simulink model "experiment_toplevel_with_tail"  (R2016a)
settings: Solver=ode15s  StartTime=0.0  StopTime=8  MaxStep=1e-2  RelTol=1e-4
PreLoadFcn:
  | minitaurParameters
values from neighbouring files (symbols this model uses):
  angular_ctrl_d = 1    [minitaurParameters.m]
  angular_ctrl_i = 1    [minitaurParameters.m]
  angular_ctrl_p = 100    [minitaurParameters.m]
  enc_zero_IA = -1.25*pi    (= -3.92699081699)    [minitaurParameters.m]
  enc_zero_IB = -0.25*pi    (= -0.785398163397)    [minitaurParameters.m]
  enc_zero_IIA = 1.25*pi    (= 3.92699081699)    [minitaurParameters.m]
  enc_zero_IIB = 1.25*pi    (= 3.92699081699)    [minitaurParameters.m]
  enc_zero_IIIA = 0.5*pi    (= 1.57079632679)    [minitaurParameters.m]
  enc_zero_IIIB = 1.5*pi    (= 4.71238898038)    [minitaurParameters.m]
  enc_zero_IVA = -0.25*pi    (= -0.785398163397)    [minitaurParameters.m]
  enc_zero_IVB = 0.5*pi    (= 1.57079632679)    [minitaurParameters.m]
  enc_zero_tail = 0    [minitaurParameters.m]
  fore_lag = fore_lag_vals(j)    [experiment1.m]    (also in experiment1_parfor_accelerator.m = 0; minitaurParameters.m = 0.45)
  ground_frame_depth = 0.5    [minitaurParameters.m]
  ground_length = 100    [minitaurParameters.m]
  ground_width = 10    [minitaurParameters.m]
  init_theta_IA = -pi/4    (= -0.785398163397)    [minitaurParameters.m]
  init_theta_IB = pi/4    (= 0.785398163397)    [minitaurParameters.m]
  init_theta_IIA = -pi/4    (= -0.785398163397)    [minitaurParameters.m]
  init_theta_IIB = pi/4    (= 0.785398163397)    [minitaurParameters.m]
  init_theta_IIIA = -pi/4    (= -0.785398163397)    [minitaurParameters.m]
  init_theta_IIIB = pi/4    (= 0.785398163397)    [minitaurParameters.m]
  init_theta_IVA = -pi/4    (= -0.785398163397)    [minitaurParameters.m]
  init_theta_IVB = pi/4    (= 0.785398163397)    [minitaurParameters.m]
  init_theta_tail = 0    [minitaurParameters.m]
  l1 = 100e-3    (= 0.1)    [minitaurParameters.m]
  l2 = 200e-3    (= 0.2)    [minitaurParameters.m]
  leg_joint_radius = 3e-3    (= 0.003)    [minitaurParameters.m]
  lr_sync = 1    [experiment1.m]    (also in experiment1_parfor_accelerator.m; minitaurParameters.m = 0)
  model = 'experiment_toplevel'    [experiment1_parfor_accelerator.m]
  period = period_vals(i)    [experiment1.m]    (also in experiment1_parfor_accelerator.m = 1.5; minitaurParameters.m = 0.33)
  phi_0 = 0.5*asin(l1/l2)    [experiment1.m]    (also in experiment1_parfor_accelerator.m; minitaurParameters.m)
  r_0 = l2    [experiment1.m]    (also in experiment1_parfor_accelerator.m; minitaurParameters.m = 0.2)
  r_x = 0.3*l1    [experiment1.m]    (also in experiment1_parfor_accelerator.m = 0.5*l1; minitaurParameters.m = 0.05)
  r_y = 0.2*l1    [experiment1.m]    (also in experiment1_parfor_accelerator.m = 0.3*l1; minitaurParameters.m = 0.03)
  radial_ctrl_d = 1    [minitaurParameters.m]
  radial_ctrl_i = 1    [minitaurParameters.m]
  radial_ctrl_p = 80    [minitaurParameters.m]
  safety_limit = 10e-3    (= 0.01)    [minitaurParameters.m]
undefined symbols (not defined in the file or in its folder): Axis, Fn, minitaurParams, r_stance, r_swing, stance_frac, X, Y, Z
undefined symbols (not defined in the file): leg_joint_fric_bw, leg_joint_mu_k, leg_joint_mu_s, leg_joint_vel_thresh, motor_kt, motor_kv, motor_r, motor_torque_sat
libraries: sm_lib x488, fl_lib x132, nesl_utility x34, Contact_Forces_Lib x28, simulink x20
(part 14 of 14)

== system experiment_toplevel_with_tail/GR Minitaur/minitaur_motor_module_IVB/DYS_BLDC_86x10_BE8108_12/DYS_BLDC_86x10_BE8108_12_stator_1_RIGID ==
  ReferenceFrame : sm_lib/Frames and Transforms/Reference Frame
  Solid : sm_lib/Body Elements/Solid  InertiaType=Custom  Mass=minitaurParams.Solid(6).mass  MassUnits=kg  CenterOfMass=minitaurParams.Solid(6).CoM  CenterOfMassUnits=mm  MomentsOfInertia=minitaurParams.Solid(6).MoI  MomentsOfInertiaUnits=kg*mm^2  ProductsOfInertia=minitaurParams.Solid(6).PoI  ProductsOfInertiaUnits=kg*mm^2  DensityBased=on  Density=1000  DensityUnits=kg/(m^3)  DoExposeReferenceFrame=on  SerializedFrames=<Frames/>  GraphicType=FromGeometry  MarkerShape=Sphere  MarkerSize=10  GraphicVisPropType=SimpleVisualProperties  GraphicDiffuseColor=minitaurParams.Solid(6).color  GraphicSpecularColor=[0.5 0.5 0.5 1.0]  GraphicAmbientColor=[0.15 0.15 0.15 1.0]  GraphicEmissiveColor=[0.0 0.0 0.0 1.0]  GraphicShininess=75  GraphicOpacity=minitaurParams.Solid(6).opacity  GeometryShape=FromFile  RectangleSize=[1 1]  RectangleSizeUnits=m  BrickDimensions=[1 1 1]  BrickDimensionUnits=m  CylinderRadius=1  CylinderRadiusUnits=m  CylinderLength=1  CylinderLengthUnits=m  SphereRadius=1  SphereRadiusUnits=m  EllipsoidRadii=[1 1 1]  EllipsoidRadiiUnits=m  ExtrusionCrossSection=[1 1; -1 1; -1 -1; 1 -1]  ExtrusionCrossSectionUnits=m  ExtrusionLength=1  ExtrusionLengthUnits=m  PolygonNumSides=3  PolygonOuterRadius=1  PolygonOuterRadiusUnits=m  ExtGeomFileType=STEP  ExtGeomFileName=model/DYS-BLDC-86x10-BE8108-12-stator_Default_sldprt.STEP  ExtGeomFileUnits=m  RevolutionCrossSection=[1 1; 1 -1; 2 -1; 2 1]  RevolutionCrossSectionUnits=m  RevolutionExtent=Full  RevolutionAngle=180  RevolutionAngleUnits=deg
  Transform : sm_lib/Frames and Transforms/Rigid Transform  TranslationMethod=Cartesian  TranslationLengthUnit=mm  TranslationStandardAxis=+Z  TranslationStandardOffset=0  TranslationCartesianOffset=minitaurParams.RigidTransform(17).translation  TranslationROffset=0  TranslationROffsetUnits=m  TranslationZOffset=0  TranslationZOffsetUnits=m  TranslationThetaOffset=0  TranslationThetaOffsetUnits=deg  RotationMethod=ArbitraryAxis  RotationAngleUnits=rad  RotationStandardAxis=+Z  RotationAngle=minitaurParams.RigidTransform(17).angle  RotationArbitraryAxis=minitaurParams.RigidTransform(17).axis  FollAlignAxisA=+X  BaseAlignAxisA=+Y  FollAlignAxisB=+Y  BaseAlignAxisB=+Z  RotationSequenceAxes=FollowerAxes  RotationSequence=XYX  RotationSequenceAngles=[0 0 0]  RotationSequenceAnglesUnits=deg  RotationMatrix=[1 0 0; 0 1 0; 0 0 1]
  Transform1 : sm_lib/Frames and Transforms/Rigid Transform  TranslationMethod=Cartesian  TranslationLengthUnit=mm  TranslationStandardAxis=+Z  TranslationStandardOffset=0  TranslationCartesianOffset=minitaurParams.RigidTransform(19).translation  TranslationROffset=0  TranslationROffsetUnits=m  TranslationZOffset=0  TranslationZOffsetUnits=m  TranslationThetaOffset=0  TranslationThetaOffsetUnits=deg  RotationMethod=ArbitraryAxis  RotationAngleUnits=rad  RotationStandardAxis=+Z  RotationAngle=minitaurParams.RigidTransform(19).angle  RotationArbitraryAxis=minitaurParams.RigidTransform(19).axis  FollAlignAxisA=+X  BaseAlignAxisA=+Y  FollAlignAxisB=+Y  BaseAlignAxisB=+Z  RotationSequenceAxes=FollowerAxes  RotationSequence=XYX  RotationSequenceAngles=[0 0 0]  RotationSequenceAnglesUnits=deg  RotationMatrix=[1 0 0; 0 1 0; 0 0 1]
  Transform2 : sm_lib/Frames and Transforms/Rigid Transform  TranslationMethod=Cartesian  TranslationLengthUnit=mm  TranslationStandardAxis=+Z  TranslationStandardOffset=0  TranslationCartesianOffset=minitaurParams.RigidTransform(26).translation  TranslationROffset=0  TranslationROffsetUnits=m  TranslationZOffset=0  TranslationZOffsetUnits=m  TranslationThetaOffset=0  TranslationThetaOffsetUnits=deg  RotationMethod=ArbitraryAxis  RotationAngleUnits=rad  RotationStandardAxis=+Z  RotationAngle=minitaurParams.RigidTransform(26).angle  RotationArbitraryAxis=minitaurParams.RigidTransform(26).axis  FollAlignAxisA=+X  BaseAlignAxisA=+Y  FollAlignAxisB=+Y  BaseAlignAxisB=+Z  RotationSequenceAxes=FollowerAxes  RotationSequence=XYX  RotationSequenceAngles=[0 0 0]  RotationSequenceAnglesUnits=deg  RotationMatrix=[1 0 0; 0 1 0; 0 0 1]
  Transform3 : sm_lib/Frames and Transforms/Rigid Transform  TranslationMethod=Cartesian  TranslationLengthUnit=mm  TranslationStandardAxis=+Z  TranslationStandardOffset=0  TranslationCartesianOffset=minitaurParams.RigidTransform(62).translation  TranslationROffset=0  TranslationROffsetUnits=m  TranslationZOffset=0  TranslationZOffsetUnits=m  TranslationThetaOffset=0  TranslationThetaOffsetUnits=deg  RotationMethod=ArbitraryAxis  RotationAngleUnits=rad  RotationStandardAxis=+Z  RotationAngle=minitaurParams.RigidTransform(62).angle  RotationArbitraryAxis=minitaurParams.RigidTransform(62).axis  FollAlignAxisA=+X  BaseAlignAxisA=+Y  FollAlignAxisB=+Y  BaseAlignAxisB=+Z  RotationSequenceAxes=FollowerAxes  RotationSequence=XYX  RotationSequenceAngles=[0 0 0]  RotationSequenceAnglesUnits=deg  RotationMatrix=[1 0 0; 0 1 0; 0 0 1]
  F2 : PMIOPort  Port=1  Side=Left
  F3 : PMIOPort  Port=2  Side=Left
  F : PMIOPort  Port=3  Side=Left
  F1 : PMIOPort  Port=4  Side=Right
  connections:
  ReferenceFrame/RConn1 -- Solid/RConn1 -- Transform/LConn1 -- Transform1/LConn1 -- Transform2/LConn1 -- Transform3/LConn1
  Transform/RConn1 -- F/RConn1
  Transform1/RConn1 -- F1/RConn1
  Transform2/RConn1 -- F2/RConn1
  Transform3/RConn1 -- F3/RConn1

== system experiment_toplevel_with_tail/GR Minitaur/minitaur_motor_module_Tail/DYS_BLDC_86x10_BE8108_12/BLDC Model ==
  Desired Torque  [Nm] : Inport
  Velocity [rad/s] : Inport  Port=2
  Constant : Constant  Value=torque_sat
  Constant1 : Constant  Value=-torque_sat
  Gain : Gain  Gain=1/kt
  Gain1 : Gain  Gain=r
  Math Function : Math  Operator=square  SaturateOnIntegerOverflow=on
  Saturation Dynamic : simulink/Discontinuities/Saturation Dynamic  OutMin=[]  OutMax=[]  OutDataTypeStr=Inherit: Same as second input  OutDataType=fixdt(1, 16)  OutScaling=2^-10  DoSatur=off
  Terminator : Terminator
  Transfer Fcn : TransferFcn  Denominator=[timeconst 1]
  Torque [N*m] : Outport
  Ploss [W] : Outport  Port=2
  wires:
  Desired Torque  [Nm]/1 -> Transfer Fcn/1
  Math Function/1 -> Gain1/1
  Gain/1 -> Math Function/1
  Gain1/1 -> Ploss [W]/1
  Velocity [rad/s]/1 -> Terminator/1
  Transfer Fcn/1 -> Saturation Dynamic/2
  Saturation Dynamic/1 -> Gain/1, Torque [N*m]/1
  Constant/1 -> Saturation Dynamic/1
  Constant1/1 -> Saturation Dynamic/3

== system experiment_toplevel_with_tail/GR Minitaur/minitaur_motor_module_Tail/DYS_BLDC_86x10_BE8108_12/DYS_BLDC_86x10_BE8108_12_rotor_1_RIGID ==
  ReferenceFrame : sm_lib/Frames and Transforms/Reference Frame
  Solid : sm_lib/Body Elements/Solid  InertiaType=Custom  Mass=minitaurParams.Solid(7).mass  MassUnits=kg  CenterOfMass=minitaurParams.Solid(7).CoM  CenterOfMassUnits=mm  MomentsOfInertia=minitaurParams.Solid(7).MoI  MomentsOfInertiaUnits=kg*mm^2  ProductsOfInertia=minitaurParams.Solid(7).PoI  ProductsOfInertiaUnits=kg*mm^2  DensityBased=on  Density=1000  DensityUnits=kg/(m^3)  DoExposeReferenceFrame=on  SerializedFrames=<Frames/>  GraphicType=FromGeometry  MarkerShape=Sphere  MarkerSize=10  GraphicVisPropType=SimpleVisualProperties  GraphicDiffuseColor=minitaurParams.Solid(7).color  GraphicSpecularColor=[0.5 0.5 0.5 1.0]  GraphicAmbientColor=[0.15 0.15 0.15 1.0]  GraphicEmissiveColor=[0.0 0.0 0.0 1.0]  GraphicShininess=75  GraphicOpacity=minitaurParams.Solid(7).opacity  GeometryShape=FromFile  RectangleSize=[1 1]  RectangleSizeUnits=m  BrickDimensions=[1 1 1]  BrickDimensionUnits=m  CylinderRadius=1  CylinderRadiusUnits=m  CylinderLength=1  CylinderLengthUnits=m  SphereRadius=1  SphereRadiusUnits=m  EllipsoidRadii=[1 1 1]  EllipsoidRadiiUnits=m  ExtrusionCrossSection=[1 1; -1 1; -1 -1; 1 -1]  ExtrusionCrossSectionUnits=m  ExtrusionLength=1  ExtrusionLengthUnits=m  PolygonNumSides=3  PolygonOuterRadius=1  PolygonOuterRadiusUnits=m  ExtGeomFileType=STEP  ExtGeomFileName=model/DYS-BLDC-86x10-BE8108-12-rotor_Default_sldprt.STEP  ExtGeomFileUnits=m  RevolutionCrossSection=[1 1; 1 -1; 2 -1; 2 1]  RevolutionCrossSectionUnits=m  RevolutionExtent=Full  RevolutionAngle=180  RevolutionAngleUnits=deg
  Transform : sm_lib/Frames and Transforms/Rigid Transform  TranslationMethod=Cartesian  TranslationLengthUnit=mm  TranslationStandardAxis=+Z  TranslationStandardOffset=0  TranslationCartesianOffset=minitaurParams.RigidTransform(20).translation  TranslationROffset=0  TranslationROffsetUnits=m  TranslationZOffset=0  TranslationZOffsetUnits=m  TranslationThetaOffset=0  TranslationThetaOffsetUnits=deg  RotationMethod=ArbitraryAxis  RotationAngleUnits=rad  RotationStandardAxis=+Z  RotationAngle=minitaurParams.RigidTransform(20).angle  RotationArbitraryAxis=minitaurParams.RigidTransform(20).axis  FollAlignAxisA=+X  BaseAlignAxisA=+Y  FollAlignAxisB=+Y  BaseAlignAxisB=+Z  RotationSequenceAxes=FollowerAxes  RotationSequence=XYX  RotationSequenceAngles=[0 0 0]  RotationSequenceAnglesUnits=deg  RotationMatrix=[1 0 0; 0 1 0; 0 0 1]
  Transform1 : sm_lib/Frames and Transforms/Rigid Transform  TranslationMethod=Cartesian  TranslationLengthUnit=mm  TranslationStandardAxis=+Z  TranslationStandardOffset=0  TranslationCartesianOffset=[0,30,0]  TranslationROffset=0  TranslationROffsetUnits=m  TranslationZOffset=0  TranslationZOffsetUnits=m  TranslationThetaOffset=0  TranslationThetaOffsetUnits=deg  RotationMethod=ArbitraryAxis  RotationAngleUnits=rad  RotationStandardAxis=+Z  RotationAngle=0  RotationArbitraryAxis=[0,1,0]  FollAlignAxisA=+X  BaseAlignAxisA=+Y  FollAlignAxisB=+Y  BaseAlignAxisB=+Z  RotationSequenceAxes=FollowerAxes  RotationSequence=XYX  RotationSequenceAngles=[0 0 0]  RotationSequenceAnglesUnits=deg  RotationMatrix=[1 0 0; 0 1 0; 0 0 1]
  F1 : PMIOPort  Port=1  Side=Left
  F : PMIOPort  Port=2  Side=Left
  connections:
  Transform/LConn1 -- Transform1/LConn1 -- ReferenceFrame/RConn1 -- Solid/RConn1
  Transform/RConn1 -- F/RConn1
  Transform1/RConn1 -- F1/RConn1

== system experiment_toplevel_with_tail/GR Minitaur/minitaur_motor_module_Tail/DYS_BLDC_86x10_BE8108_12/DYS_BLDC_86x10_BE8108_12_stator_1_RIGID ==
  ReferenceFrame : sm_lib/Frames and Transforms/Reference Frame
  Solid : sm_lib/Body Elements/Solid  InertiaType=Custom  Mass=minitaurParams.Solid(6).mass  MassUnits=kg  CenterOfMass=minitaurParams.Solid(6).CoM  CenterOfMassUnits=mm  MomentsOfInertia=minitaurParams.Solid(6).MoI  MomentsOfInertiaUnits=kg*mm^2  ProductsOfInertia=minitaurParams.Solid(6).PoI  ProductsOfInertiaUnits=kg*mm^2  DensityBased=on  Density=1000  DensityUnits=kg/(m^3)  DoExposeReferenceFrame=on  SerializedFrames=<Frames/>  GraphicType=FromGeometry  MarkerShape=Sphere  MarkerSize=10  GraphicVisPropType=SimpleVisualProperties  GraphicDiffuseColor=minitaurParams.Solid(6).color  GraphicSpecularColor=[0.5 0.5 0.5 1.0]  GraphicAmbientColor=[0.15 0.15 0.15 1.0]  GraphicEmissiveColor=[0.0 0.0 0.0 1.0]  GraphicShininess=75  GraphicOpacity=minitaurParams.Solid(6).opacity  GeometryShape=FromFile  RectangleSize=[1 1]  RectangleSizeUnits=m  BrickDimensions=[1 1 1]  BrickDimensionUnits=m  CylinderRadius=1  CylinderRadiusUnits=m  CylinderLength=1  CylinderLengthUnits=m  SphereRadius=1  SphereRadiusUnits=m  EllipsoidRadii=[1 1 1]  EllipsoidRadiiUnits=m  ExtrusionCrossSection=[1 1; -1 1; -1 -1; 1 -1]  ExtrusionCrossSectionUnits=m  ExtrusionLength=1  ExtrusionLengthUnits=m  PolygonNumSides=3  PolygonOuterRadius=1  PolygonOuterRadiusUnits=m  ExtGeomFileType=STEP  ExtGeomFileName=model/DYS-BLDC-86x10-BE8108-12-stator_Default_sldprt.STEP  ExtGeomFileUnits=m  RevolutionCrossSection=[1 1; 1 -1; 2 -1; 2 1]  RevolutionCrossSectionUnits=m  RevolutionExtent=Full  RevolutionAngle=180  RevolutionAngleUnits=deg
  Transform : sm_lib/Frames and Transforms/Rigid Transform  TranslationMethod=Cartesian  TranslationLengthUnit=mm  TranslationStandardAxis=+Z  TranslationStandardOffset=0  TranslationCartesianOffset=minitaurParams.RigidTransform(17).translation  TranslationROffset=0  TranslationROffsetUnits=m  TranslationZOffset=0  TranslationZOffsetUnits=m  TranslationThetaOffset=0  TranslationThetaOffsetUnits=deg  RotationMethod=ArbitraryAxis  RotationAngleUnits=rad  RotationStandardAxis=+Z  RotationAngle=minitaurParams.RigidTransform(17).angle  RotationArbitraryAxis=minitaurParams.RigidTransform(17).axis  FollAlignAxisA=+X  BaseAlignAxisA=+Y  FollAlignAxisB=+Y  BaseAlignAxisB=+Z  RotationSequenceAxes=FollowerAxes  RotationSequence=XYX  RotationSequenceAngles=[0 0 0]  RotationSequenceAnglesUnits=deg  RotationMatrix=[1 0 0; 0 1 0; 0 0 1]
  Transform1 : sm_lib/Frames and Transforms/Rigid Transform  TranslationMethod=Cartesian  TranslationLengthUnit=mm  TranslationStandardAxis=+Z  TranslationStandardOffset=0  TranslationCartesianOffset=minitaurParams.RigidTransform(19).translation  TranslationROffset=0  TranslationROffsetUnits=m  TranslationZOffset=0  TranslationZOffsetUnits=m  TranslationThetaOffset=0  TranslationThetaOffsetUnits=deg  RotationMethod=ArbitraryAxis  RotationAngleUnits=rad  RotationStandardAxis=+Z  RotationAngle=minitaurParams.RigidTransform(19).angle  RotationArbitraryAxis=minitaurParams.RigidTransform(19).axis  FollAlignAxisA=+X  BaseAlignAxisA=+Y  FollAlignAxisB=+Y  BaseAlignAxisB=+Z  RotationSequenceAxes=FollowerAxes  RotationSequence=XYX  RotationSequenceAngles=[0 0 0]  RotationSequenceAnglesUnits=deg  RotationMatrix=[1 0 0; 0 1 0; 0 0 1]
  Transform2 : sm_lib/Frames and Transforms/Rigid Transform  TranslationMethod=Cartesian  TranslationLengthUnit=mm  TranslationStandardAxis=+Z  TranslationStandardOffset=0  TranslationCartesianOffset=minitaurParams.RigidTransform(26).translation  TranslationROffset=0  TranslationROffsetUnits=m  TranslationZOffset=0  TranslationZOffsetUnits=m  TranslationThetaOffset=0  TranslationThetaOffsetUnits=deg  RotationMethod=ArbitraryAxis  RotationAngleUnits=rad  RotationStandardAxis=+Z  RotationAngle=minitaurParams.RigidTransform(26).angle  RotationArbitraryAxis=minitaurParams.RigidTransform(26).axis  FollAlignAxisA=+X  BaseAlignAxisA=+Y  FollAlignAxisB=+Y  BaseAlignAxisB=+Z  RotationSequenceAxes=FollowerAxes  RotationSequence=XYX  RotationSequenceAngles=[0 0 0]  RotationSequenceAnglesUnits=deg  RotationMatrix=[1 0 0; 0 1 0; 0 0 1]
  Transform3 : sm_lib/Frames and Transforms/Rigid Transform  TranslationMethod=Cartesian  TranslationLengthUnit=mm  TranslationStandardAxis=+Z  TranslationStandardOffset=0  TranslationCartesianOffset=[0,0,0]  TranslationROffset=0  TranslationROffsetUnits=m  TranslationZOffset=0  TranslationZOffsetUnits=m  TranslationThetaOffset=0  TranslationThetaOffsetUnits=deg  RotationMethod=ArbitraryAxis  RotationAngleUnits=rad  RotationStandardAxis=+Z  RotationAngle=minitaurParams.RigidTransform(62).angle  RotationArbitraryAxis=minitaurParams.RigidTransform(62).axis  FollAlignAxisA=+X  BaseAlignAxisA=+Y  FollAlignAxisB=+Y  BaseAlignAxisB=+Z  RotationSequenceAxes=FollowerAxes  RotationSequence=XYX  RotationSequenceAngles=[0 0 0]  RotationSequenceAnglesUnits=deg  RotationMatrix=[1 0 0; 0 1 0; 0 0 1]
  F2 : PMIOPort  Port=1  Side=Left
  F3 : PMIOPort  Port=2  Side=Left
  F : PMIOPort  Port=3  Side=Left
  F1 : PMIOPort  Port=4  Side=Right
  connections:
  ReferenceFrame/RConn1 -- Transform2/LConn1 -- Transform3/LConn1 -- Transform/LConn1 -- Transform1/LConn1 -- Solid/RConn1
  Transform/RConn1 -- F/RConn1
  Transform1/RConn1 -- F1/RConn1
  Transform2/RConn1 -- F2/RConn1
  Transform3/RConn1 -- F3/RConn1

== matlab function experiment_toplevel_with_tail/Controller/Subsystem5/Minitaur Leg Actuator Coordinates to Configuration Coordinates1 ==
  data: a output; q input
function a = legActToConfig(q)
% Converts from actuator coordinates q = [theta_A theta_B] to leg
% configuration a = [alpha beta].

    a = [pi 0]' + 0.5*[1 1; 1 -1]*q;

end

== matlab function experiment_toplevel_with_tail/Controller/Subsystem5/Minitaur Leg Inverse Dynamics ==
  data: f input; tau output; a input; l1 input; l2 input
function tau = legInvDynamics(f,a,l1,l2)
% Computes the actuator torques corresponding to the desired end-effector
% force. Implements tau = J'f, where J is the J' is the leg jacobian
% transpose.

    % Compute leg jacobian
    B = a(2);
    dRdB = l1*sin(B)-(l1^2*sin(B)*cos(B))/sqrt(l2^2-(l1*sin(B))^2);
%     J = 0.5*[1 1; dRdB -1];

    J = 0.5*[1 1; -dRdB 1];
    
    % Compute actuator torques
    tau = J'*f;
    
end

== matlab function experiment_toplevel_with_tail/Controller/Subsystem5/Minitaur Leg Polar Forward Kinematics ==
  data: a input; p output; l1 input; l2 input
function p = legPolarFK(a,l1,l2)
% Computes the forward kinematics for the minitaur leg in polar
% coordinates.
% a = [alpha beta] are the leg configuration parameters

    p = zeros(2,1);
    p(1) = a(1);
    p(2) = sqrt(l2^2-(l1*sin(a(2)))^2)-l1*cos(a(2));
    
end

== matlab function experiment_toplevel_with_tail/Controller/Subsystem1/Minitaur Leg Actuator Coordinates to Configuration Coordinates1 ==
  data: a output; q input
function a = legActToConfig(q)
% Converts from actuator coordinates q = [theta_A theta_B] to leg
% configuration a = [alpha beta].

    a = [pi 0]' + 0.5*[1 1; 1 -1]*q;

end

== matlab function experiment_toplevel_with_tail/Controller/Subsystem1/Minitaur Leg Inverse Dynamics ==
  data: f input; tau output; a input; l1 input; l2 input
function tau = legInvDynamics(f,a,l1,l2)
% Computes the actuator torques corresponding to the desired end-effector
% force. Implements tau = J'f, where J is the J' is the leg jacobian
% transpose.

    % Compute leg jacobian
    B = a(2);
    dRdB = l1*sin(B)-(l1^2*sin(B)*cos(B))/sqrt(l2^2-(l1*sin(B))^2);
%     J = 0.5*[1 1; dRdB -1];

    J = 0.5*[1 1; -dRdB 1];
    
    % Compute actuator torques
    tau = J'*f;
    
end

== matlab function experiment_toplevel_with_tail/Controller/Subsystem1/Minitaur Leg Polar Forward Kinematics ==
  data: a input; p output; l1 input; l2 input
function p = legPolarFK(a,l1,l2)
% Computes the forward kinematics for the minitaur leg in polar
% coordinates.
% a = [alpha beta] are the leg configuration parameters

    p = zeros(2,1);
    p(1) = a(1);
    p(2) = sqrt(l2^2-(l1*sin(a(2)))^2)-l1*cos(a(2));
    
end

== matlab function experiment_toplevel_with_tail/Controller/Subsystem2/Minitaur Leg Actuator Coordinates to Configuration Coordinates1 ==
  data: a output; q input
function a = legActToConfig(q)
% Converts from actuator coordinates q = [theta_A theta_B] to leg
% configuration a = [alpha beta].

    a = [pi 0]' + 0.5*[1 1; 1 -1]*q;

end

== matlab function experiment_toplevel_with_tail/Controller/Subsystem2/Minitaur Leg Inverse Dynamics ==
  data: f input; tau output; a input; l1 input; l2 input
function tau = legInvDynamics(f,a,l1,l2)
% Computes the actuator torques corresponding to the desired end-effector
% force. Implements tau = J'f, where J is the J' is the leg jacobian
% transpose.

    % Compute leg jacobian
    B = a(2);
    dRdB = l1*sin(B)-(l1^2*sin(B)*cos(B))/sqrt(l2^2-(l1*sin(B))^2);
%     J = 0.5*[1 1; dRdB -1];

    J = 0.5*[1 1; -dRdB 1];
    
    % Compute actuator torques
    tau = J'*f;
    
end

== matlab function experiment_toplevel_with_tail/Controller/Subsystem2/Minitaur Leg Polar Forward Kinematics ==
  data: a input; p output; l1 input; l2 input
function p = legPolarFK(a,l1,l2)
% Computes the forward kinematics for the minitaur leg in polar
% coordinates.
% a = [alpha beta] are the leg configuration parameters

    p = zeros(2,1);
    p(1) = a(1);
    p(2) = sqrt(l2^2-(l1*sin(a(2)))^2)-l1*cos(a(2));
    
end

== matlab function experiment_toplevel_with_tail/Controller/Subsystem3/Minitaur Leg Actuator Coordinates to Configuration Coordinates1 ==
  data: a output; q input
function a = legActToConfig(q)
% Converts from actuator coordinates q = [theta_A theta_B] to leg
% configuration a = [alpha beta].

    a = [pi 0]' + 0.5*[1 1; 1 -1]*q;

end

== matlab function experiment_toplevel_with_tail/Controller/Subsystem3/Minitaur Leg Inverse Dynamics ==
  data: f input; tau output; a input; l1 input; l2 input
function tau = legInvDynamics(f,a,l1,l2)
% Computes the actuator torques corresponding to the desired end-effector
% force. Implements tau = J'f, where J is the J' is the leg jacobian
% transpose.

    % Compute leg jacobian
    B = a(2);
    dRdB = l1*sin(B)-(l1^2*sin(B)*cos(B))/sqrt(l2^2-(l1*sin(B))^2);
%     J = 0.5*[1 1; dRdB -1];

    J = 0.5*[1 1; -dRdB 1];
    
    % Compute actuator torques
    tau = J'*f;
    
end

== matlab function experiment_toplevel_with_tail/Controller/Subsystem3/Minitaur Leg Polar Forward Kinematics ==
  data: a input; p output; l1 input; l2 input
function p = legPolarFK(a,l1,l2)
% Computes the forward kinematics for the minitaur leg in polar
% coordinates.
% a = [alpha beta] are the leg configuration parameters

    p = zeros(2,1);
    p(1) = a(1);
    p(2) = sqrt(l2^2-(l1*sin(a(2)))^2)-l1*cos(a(2));
    
end
